simulink model "Project4Simulink"  (R2020a)
settings: Solver=VariableStepAuto  StartTime=0.0  StopTime=100.0  MaxStep=0.01  RelTol=1e-3
values from neighbouring files (symbols this model uses):
  b = 0.3    [Project4.m]    (also in Project5.m = 1)
  F = 1    [Project4.m]    (also in Project5.m = 10)
  k = 20    [Project4.m]    (also in Project5.m)
  M = 1    [Project4.m]    (also in Project5.m)
settings Model: Creator=cresp  LastModifiedBy=cresp

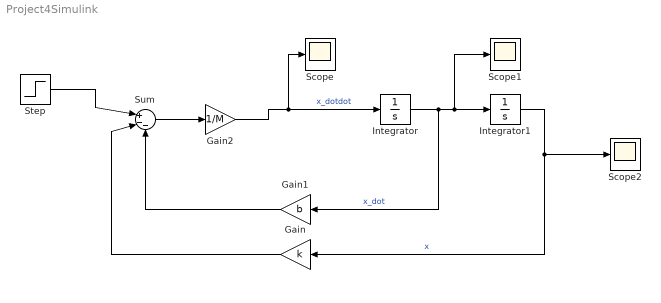
== system Project4Simulink ==
  Gain : Gain  Gain=k
  Gain1 : Gain  Gain=b
  Gain2 : Gain  Gain=1/M
  Integrator : Integrator
  Integrator1 : Integrator
  Scope : Scope
  Scope1 : Scope
  Scope2 : Scope
  Step : Step  After=F  SampleTime=0
  Sum : Sum  Inputs=|+--
  wires:
  Integrator/1 -> Gain1/1, Scope1/1, Integrator1/1  "x_dot"
  Sum/1 -> Gain2/1
  Integrator1/1 -> Gain/1, Scope2/1  "x"
  Step/1 -> Sum/1
  Gain/1 -> Sum/2
  Gain1/1 -> Sum/3
  Gain2/1 -> Scope/1, Integrator/1  "x_dotdot"
